simulink model "Project7"  (R2024a)
settings: Solver=VariableStepAuto  StartTime=0.0  StopTime=7  MaxStep=0.05  RelTol=1e-3
undefined symbols (not defined in the file): b, F, k, Kd, Ki, Kp, M
settings Model: Creator=harsh  LastModifiedBy=harsh

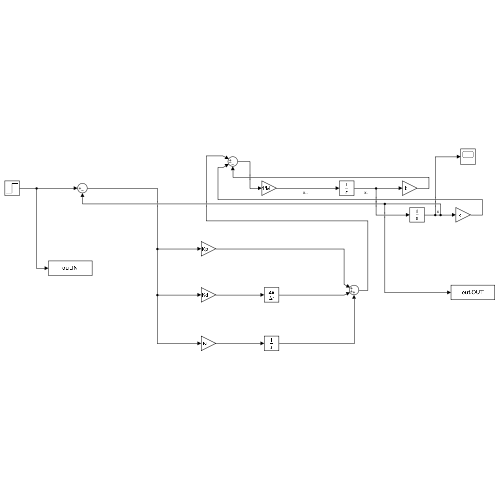
[thumbnail: Simulink's stored preview of the top-level diagram]
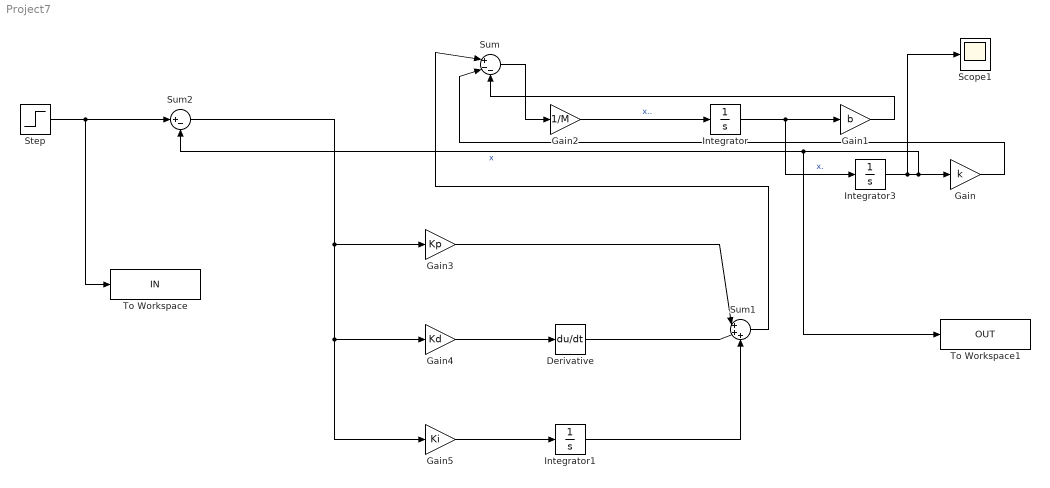
== system Project7 ==
  Derivative : Derivative
  Gain : Gain  Gain=k
  Gain1 : Gain  Gain=b
  Gain2 : Gain  Gain=1/M
  Gain3 : Gain  Gain=Kp
  Gain4 : Gain  Gain=Kd
  Gain5 : Gain  Gain=Ki
  Integrator : Integrator
  Integrator1 : Integrator
  Integrator3 : Integrator
  Scope1 : Scope
  Step : Step  After=F  SampleTime=0
  Sum : Sum  Inputs=|+--
  Sum1 : Sum  Inputs=|+++
  Sum2 : Sum  Inputs=|+-
  To Workspace : ToWorkspace  VariableName=IN  SaveFormat=Timeseries  SampleTime=-1
  To Workspace1 : ToWorkspace  VariableName=OUT  SaveFormat=Timeseries  SampleTime=-1
  wires:
  Integrator/1 -> Integrator3/1, Gain1/1  "x."
  Gain2/1 -> Integrator/1  "x.."
  Gain1/1 -> Sum/3
  Integrator3/1 -> Gain/1, To Workspace1/1, Sum2/2, Scope1/1  "x"
  Gain/1 -> Sum/2
  Sum/1 -> Gain2/1
  Gain4/1 -> Derivative/1
  Sum2/1 -> Gain5/1, Gain4/1, Gain3/1
  Integrator1/1 -> Sum1/3
  Gain5/1 -> Integrator1/1
  Derivative/1 -> Sum1/2
  Gain3/1 -> Sum1/1
  Sum1/1 -> Sum/1
  Step/1 -> To Workspace/1, Sum2/1
